simulink library "IPT_lib"  (Simulink 7.4)
settings: Solver=ode45  StartTime=0.0  StopTime=10.0  RelTol=1e-3
values from neighbouring files (symbols this model uses):
  IPTa_i_ShuntCur = mpt.Parameter    [IPT_ANALOG_CAL.m]
  IPTc_Gain_KL30 = mpt.Parameter    [IPT_ANALOG_CAL.m]
  IPTc_Gain_MSDVolt = mpt.Parameter    [IPT_ANALOG_CAL.m]
  IPTc_Gain_PCBTemp = mpt.Parameter    [IPT_ANALOG_CAL.m]
  IPTc_Gain_PosCtrVoltRef1_back = mpt.Parameter    [IPT_ANALOG_CAL.m]
  IPTc_Gain_PosCtrVoltRef1_front = mpt.Parameter    [IPT_ANALOG_CAL.m]
  IPTc_Gain_PosCtrVoltRef2_back = mpt.Parameter    [IPT_ANALOG_CAL.m]
  IPTc_Gain_PosCtrVoltRef2_front = mpt.Parameter    [IPT_ANALOG_CAL.m]
  IPTc_pct_CellInitSoc = mpt.Parameter    [IPT_INTERNAL_CAL.m]
  IPTc_t_BMUInitTemp = mpt.Parameter    [IPT_CAN_CAL.m]
  IPTc_t_MdlInitTemp = mpt.Parameter    [IPT_CAN_CAL.m]
  IPTc_t_PCBTemp_max = mpt.Parameter    [IPT_ANALOG_CAL.m]
  IPTc_t_PCBTemp_min = mpt.Parameter    [IPT_ANALOG_CAL.m]
  IPTc_v_KL30_max = mpt.Parameter    [IPT_ANALOG_CAL.m]
  IPTc_v_KL30_min = mpt.Parameter    [IPT_ANALOG_CAL.m]
  IPTc_v_MSDVolt_max = mpt.Parameter    [IPT_ANALOG_CAL.m]
  IPTc_v_MSDVolt_min = mpt.Parameter    [IPT_ANALOG_CAL.m]
  IPTc_v_PosCtrVoltRef1_back_max = mpt.Parameter    [IPT_ANALOG_CAL.m]
  IPTc_v_PosCtrVoltRef1_back_min = mpt.Parameter    [IPT_ANALOG_CAL.m]
  IPTc_v_PosCtrVoltRef1_front_max = mpt.Parameter    [IPT_ANALOG_CAL.m]
  IPTc_v_PosCtrVoltRef1_front_min = mpt.Parameter    [IPT_ANALOG_CAL.m]
  IPTc_v_PosCtrVoltRef2_back_max = mpt.Parameter    [IPT_ANALOG_CAL.m]
  IPTc_v_PosCtrVoltRef2_back_min = mpt.Parameter    [IPT_ANALOG_CAL.m]
  IPTc_v_PosCtrVoltRef2_front_max = mpt.Parameter    [IPT_ANALOG_CAL.m]
  IPTc_v_PosCtrVoltRef2_front_min = mpt.Parameter    [IPT_ANALOG_CAL.m]
  IPTf_fac_ShuntCurCorrect = mpt.Parameter    [IPT_ANALOG_CAL.m]
undefined symbols (not defined in the file or in its folder): CTC_DriveOnline_St, CTC_FastChaOnline_St, CTC_SlowChaOnline_St, IPTa_v_PCBTemp, IPTc_Gain_BMUPowSplyCur, IPTc_Gain_ShuntCur, IPTc_Gain_USample, IPTc_i_BMUPowSplyCur_max, IPTc_i_BMUPowSplyCur_min, IPTc_i_ShuntCur_max, IPTc_i_ShuntCur_min, IPTc_v_CC2_OffDnLimit, IPTc_v_CC2_OffUpLimit, IPTc_v_CC2_OnDnLimit, IPTc_v_CC2_OnUpLimit, IPTc_v_CellInitVolt, IPTc_v_SlowChalineCnctStLowLimFir, IPTc_v_SlowChalineCnctStLowLimSec, IPTc_v_SlowChalineCnctStUppLimFir, IPTc_v_SlowChalineCnctStUppLimSec, IPTc_v_SlowChalineOpenLowLim, IPTc_v_SlowChalineOpenUppLim, IPTc_v_USample_max, IPTc_v_USample_min, IPTf_t_PCBTemp, PACK_Const_BMUNumOfPack
libraries: Defined_Functionality x129
(part 2 of 3)

== system IPT_lib/IPT/ip_analog/PosCtrVoltRef1_front ==
  HLd_adc_PosCtrVoltRef1_front : Inport
  IPTd_flg_VoltFlterAlwd : Inport  Port=2
  ADC to Actual Value1 : Defined_Functionality/ADC to Actual Value1  SystemSampleTime=-1  offset=IPTc_Offset_PosCtrVoltRef1_front  gain=IPTc_Gain_PosCtrVoltRef1_front
      settings: AttributesFormatString=[OFFSET=%<offset>]\n[GAIN=%<gain>]
  Constant : Constant  Value=IPTc_v_PosCtrVoltRef1_front_max  OutDataTypeMode=single  OutDataType=fixdt(1, 16)  OutScaling=2^0  OutDataTypeStr=single
  Constant1 : Constant  Value=IPTc_v_PosCtrVoltRef1_front_min  OutDataTypeMode=single  OutDataType=fixdt(1, 16)  OutScaling=2^0  OutDataTypeStr=single
  LPF1 : Defined_Functionality/LPF  SystemSampleTime=-1  filter_gain=IPTc_flter_PosCtrVoltRef1_front
      settings: AttributesFormatString=[FILTER_GAIN=%<filter_gain>]
  Logical Operator : Logic  Operator=OR  AllPortsSameDT=off  OutDataTypeMode=boolean  LogicDataType=fixdt(0, 8)  OutDataTypeStr=boolean
  Relational Operator : RelationalOperator  Operator=>  LogicOutDataTypeMode=boolean  LogicDataType=fixdt(0, 8)  OutDataTypeStr=boolean
  Relational Operator1 : RelationalOperator  Operator=<  LogicOutDataTypeMode=boolean  LogicDataType=fixdt(0, 8)  OutDataTypeStr=boolean
  Switch14 : Switch  Criteria=u2 ~= 0  Threshold=0.5  OutDataTypeMode=single  OutDataType=sfix(16)  OutScaling=2^0  OutDataTypeStr=single
  saturation : Defined_Functionality/saturation  SystemSampleTime=-1  upper_limit=IPTc_v_PosCtrVoltRef1_front_max  lower_limit=IPTc_v_PosCtrVoltRef1_front_min
      settings: AttributesFormatString=[UPPER_LIMIT=%<upper_limit>]\n[LOWER_LIMIT=%<lower_limit>]
  signal_debug : Defined_Functionality/signal_debug  SystemSampleTime=-1  debug_switch=IPTc_dbgsw_PosCtrVoltRef1_front  debug_value=IPTc_dbgval_PosCtrVoltRef1_front
  IPTd_v_PosCtrVoltRef1_front : Outport
  IPTd_iflt_PosCtrVoltRef1_front : Outport  Port=2
  wires:
  ADC to Actual Value1/1 -> [IPTd_v_Raw], LPF1/1
  [IPTd_v_Raw] -> Switch14/3
  LPF1/1 -> Switch14/1
  Switch14/1 -> Relational Operator1/1, Relational Operator/1, saturation/1
  IPTd_flg_VoltFlterAlwd/1 -> Switch14/2
  Constant/1 -> Relational Operator/2
  Constant1/1 -> Relational Operator1/2
  Relational Operator/1 -> Logical Operator/1
  Relational Operator1/1 -> Logical Operator/2
  saturation/1 -> signal_debug/1
  HLd_adc_PosCtrVoltRef1_front/1 -> ADC to Actual Value1/1
  Logical Operator/1 -> IPTd_iflt_PosCtrVoltRef1_front/1  "IPTd_iflt_PosCtrVoltRef1_front"
  signal_debug/1 -> IPTd_v_PosCtrVoltRef1_front/1  "IPTd_v_PosCtrVoltRef1_front"

== system IPT_lib/IPT/ip_analog/PosCtrVoltRef2_back ==
  HLd_adc_PosCtrVoltRef2_back : Inport
  IPTd_flg_VoltFlterAlwd : Inport  Port=2
  ADC to Actual Value1 : Defined_Functionality/ADC to Actual Value1  SystemSampleTime=-1  offset=IPTc_Offset_PosCtrVoltRef2_back  gain=IPTc_Gain_PosCtrVoltRef2_back
      settings: AttributesFormatString=[OFFSET=%<offset>]\n[GAIN=%<gain>]
  Constant : Constant  Value=IPTc_v_PosCtrVoltRef2_back_max  OutDataTypeMode=single  OutDataType=fixdt(1, 16)  OutScaling=2^0  OutDataTypeStr=single
  Constant1 : Constant  Value=IPTc_v_PosCtrVoltRef2_back_min  OutDataTypeMode=single  OutDataType=fixdt(1, 16)  OutScaling=2^0  OutDataTypeStr=single
  LPF1 : Defined_Functionality/LPF  SystemSampleTime=-1  filter_gain=IPTc_flter_PosCtrVoltRef2_back
      settings: AttributesFormatString=[FILTER_GAIN=%<filter_gain>]
  Logical Operator : Logic  Operator=OR  AllPortsSameDT=off  OutDataTypeMode=boolean  LogicDataType=fixdt(0, 8)  OutDataTypeStr=boolean
  Relational Operator : RelationalOperator  Operator=>  LogicOutDataTypeMode=boolean  LogicDataType=fixdt(0, 8)  OutDataTypeStr=boolean
  Relational Operator1 : RelationalOperator  Operator=<  LogicOutDataTypeMode=boolean  LogicDataType=fixdt(0, 8)  OutDataTypeStr=boolean
  Switch14 : Switch  Criteria=u2 ~= 0  Threshold=0.5  OutDataTypeMode=single  OutDataType=sfix(16)  OutScaling=2^0  OutDataTypeStr=single
  saturation : Defined_Functionality/saturation  SystemSampleTime=-1  upper_limit=IPTc_v_PosCtrVoltRef2_back_max  lower_limit=IPTc_v_PosCtrVoltRef2_back_min
      settings: AttributesFormatString=[UPPER_LIMIT=%<upper_limit>]\n[LOWER_LIMIT=%<lower_limit>]
  signal_debug : Defined_Functionality/signal_debug  SystemSampleTime=-1  debug_switch=IPTc_dbgsw_PosCtrVoltRef2_back  debug_value=IPTc_dbgval_PosCtrVoltRef2_back
  IPTd_v_PosCtrVoltRef2_back : Outport
  IPTd_iflt_PosCtrVoltRef2_back : Outport  Port=2
  wires:
  ADC to Actual Value1/1 -> [IPTd_v_Raw], LPF1/1  "IPTd_v_PosCtrVoltRef2_back_raw"
  Switch14/1 -> Relational Operator1/1, Relational Operator/1, saturation/1
  LPF1/1 -> Switch14/1
  [IPTd_v_Raw] -> Switch14/3
  IPTd_flg_VoltFlterAlwd/1 -> Switch14/2
  Relational Operator/1 -> Logical Operator/1
  Constant/1 -> Relational Operator/2
  Constant1/1 -> Relational Operator1/2
  Relational Operator1/1 -> Logical Operator/2
  saturation/1 -> signal_debug/1
  HLd_adc_PosCtrVoltRef2_back/1 -> ADC to Actual Value1/1
  Logical Operator/1 -> IPTd_iflt_PosCtrVoltRef2_back/1  "IPTd_iflt_PosCtrVoltRef2_back"
  signal_debug/1 -> IPTd_v_PosCtrVoltRef2_back/1  "IPTd_v_PosCtrVoltRef2_back"

== system IPT_lib/IPT/ip_analog/PosCtrVoltRef2_front ==
  HLd_adc_PosCtrVoltRef2_front : Inport
  IPTd_flg_VoltFlterAlwd : Inport  Port=2
  ADC to Actual Value1 : Defined_Functionality/ADC to Actual Value1  SystemSampleTime=-1  offset=IPTc_Offset_PosCtrVoltRef2_front  gain=IPTc_Gain_PosCtrVoltRef2_front
      settings: AttributesFormatString=[OFFSET=%<offset>]\n[GAIN=%<gain>]
  Constant : Constant  Value=IPTc_v_PosCtrVoltRef2_front_max  OutDataTypeMode=single  OutDataType=fixdt(1, 16)  OutScaling=2^0  OutDataTypeStr=single
  Constant1 : Constant  Value=IPTc_v_PosCtrVoltRef2_front_min  OutDataTypeMode=single  OutDataType=fixdt(1, 16)  OutScaling=2^0  OutDataTypeStr=single
  LPF1 : Defined_Functionality/LPF  SystemSampleTime=-1  filter_gain=IPTc_flter_PosCtrVoltRef2_front
      settings: AttributesFormatString=[FILTER_GAIN=%<filter_gain>]
  Logical Operator : Logic  Operator=OR  AllPortsSameDT=off  OutDataTypeMode=boolean  LogicDataType=fixdt(0, 8)  OutDataTypeStr=boolean
  Relational Operator : RelationalOperator  Operator=>  LogicOutDataTypeMode=boolean  LogicDataType=fixdt(0, 8)  OutDataTypeStr=boolean
  Relational Operator1 : RelationalOperator  Operator=<  LogicOutDataTypeMode=boolean  LogicDataType=fixdt(0, 8)  OutDataTypeStr=boolean
  Switch14 : Switch  Criteria=u2 ~= 0  Threshold=0.5  OutDataTypeMode=single  OutDataType=sfix(16)  OutScaling=2^0  OutDataTypeStr=single
  saturation : Defined_Functionality/saturation  SystemSampleTime=-1  upper_limit=IPTc_v_PosCtrVoltRef2_front_max  lower_limit=IPTc_v_PosCtrVoltRef2_front_min
      settings: AttributesFormatString=[UPPER_LIMIT=%<upper_limit>]\n[LOWER_LIMIT=%<lower_limit>]
  signal_debug : Defined_Functionality/signal_debug  SystemSampleTime=-1  debug_switch=IPTc_dbgsw_PosCtrVoltRef2_front  debug_value=IPTc_dbgval_PosCtrVoltRef2_front
  IPTd_v_PosCtrVoltRef2_front : Outport
  IPTd_iflt_PosCtrVoltRef2_front : Outport  Port=2
  wires:
  ADC to Actual Value1/1 -> [IPTd_v_Raw], LPF1/1  "IPTd_v_PosCtrVoltRef2_front_raw"
  Switch14/1 -> Relational Operator1/1, Relational Operator/1, saturation/1
  LPF1/1 -> Switch14/1
  [IPTd_v_Raw] -> Switch14/3
  IPTd_flg_VoltFlterAlwd/1 -> Switch14/2
  Constant/1 -> Relational Operator/2
  Relational Operator1/1 -> Logical Operator/2
  Relational Operator/1 -> Logical Operator/1
  Constant1/1 -> Relational Operator1/2
  saturation/1 -> signal_debug/1
  signal_debug/1 -> IPTd_v_PosCtrVoltRef2_front/1  "IPTd_v_PosCtrVoltRef2_front"
  Logical Operator/1 -> IPTd_iflt_PosCtrVoltRef2_front/1  "IPTd_iflt_PosCtrVoltRef2_front"
  HLd_adc_PosCtrVoltRef2_front/1 -> ADC to Actual Value1/1

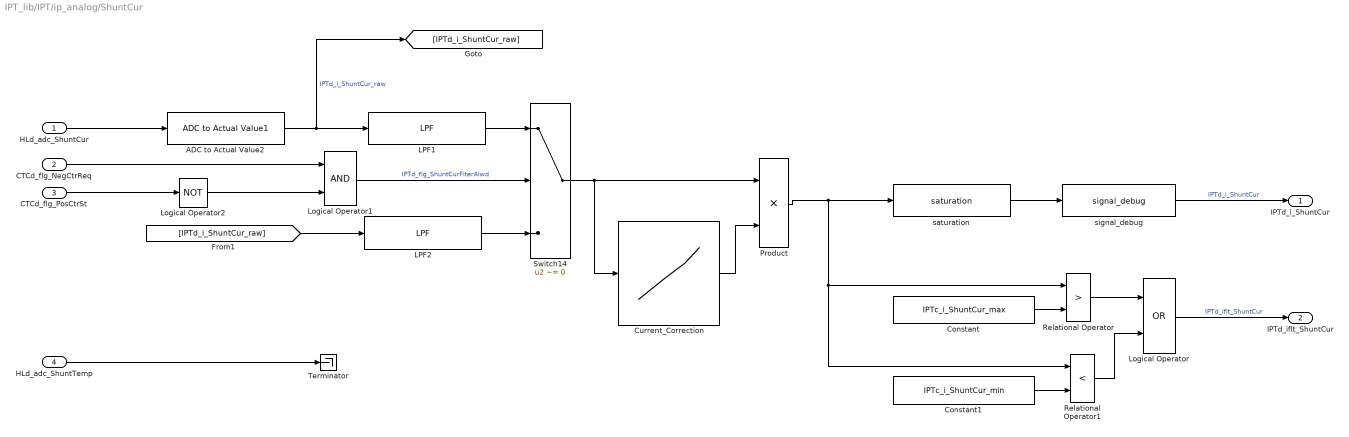
== system IPT_lib/IPT/ip_analog/ShuntCur ==
  HLd_adc_ShuntCur : Inport
  CTCd_flg_NegCtrReq : Inport  Port=2
  CTCd_flg_PosCtrSt : Inport  Port=3
  HLd_adc_ShuntTemp : Inport  Port=4
  ADC to Actual Value2 : Defined_Functionality/ADC to Actual Value1  SystemSampleTime=-1  offset=IPTc_Offset_ShuntCur  gain=IPTc_Gain_ShuntCur
      settings: AttributesFormatString=[OFFSET=%<offset>]\n[GAIN=%<gain>]
  Constant : Constant  Value=IPTc_i_ShuntCur_max  OutDataTypeMode=single  OutDataType=fixdt(1, 16)  OutScaling=2^0  OutDataTypeStr=single
  Constant1 : Constant  Value=IPTc_i_ShuntCur_min  OutDataTypeMode=single  OutDataType=fixdt(1, 16)  OutScaling=2^0  OutDataTypeStr=single
  Current_Correction : Lookup  InputValues=IPTa_i_ShuntCur  Table=IPTf_fac_ShuntCurCorrect  OutDataType=fixdt(1, 16)  OutScaling=2^0
  LPF1 : Defined_Functionality/LPF  SystemSampleTime=-1  filter_gain=IPTc_flter_ShuntCur1
      settings: AttributesFormatString=[FILTER_GAIN=%<filter_gain>]
  LPF2 : Defined_Functionality/LPF  SystemSampleTime=-1  filter_gain=IPTc_flter_ShuntCur2
      settings: AttributesFormatString=[FILTER_GAIN=%<filter_gain>]
  Logical Operator : Logic  Operator=OR  AllPortsSameDT=off  OutDataTypeMode=boolean  LogicDataType=fixdt(0, 8)  OutDataTypeStr=boolean
  Logical Operator1 : Logic  AllPortsSameDT=off  OutDataTypeMode=boolean  LogicDataType=fixdt(0, 8)  OutDataTypeStr=boolean
  Logical Operator2 : Logic  Operator=NOT  AllPortsSameDT=off  OutDataTypeMode=boolean  LogicDataType=fixdt(0, 8)  OutDataTypeStr=boolean
  Product : Product  OutDataType=fixdt(1, 16)  OutScaling=2^0  RndMeth=Zero
  Relational Operator : RelationalOperator  Operator=>  LogicOutDataTypeMode=boolean  LogicDataType=fixdt(0, 8)  OutDataTypeStr=boolean
  Relational Operator1 : RelationalOperator  Operator=<  LogicOutDataTypeMode=boolean  LogicDataType=fixdt(0, 8)  OutDataTypeStr=boolean
  Switch14 : Switch  Criteria=u2 ~= 0  Threshold=0.5  OutDataTypeMode=single  OutDataType=sfix(16)  OutScaling=2^0  OutDataTypeStr=single
  Terminator : Terminator
  saturation : Defined_Functionality/saturation  SystemSampleTime=-1  upper_limit=IPTc_i_ShuntCur_max  lower_limit=IPTc_i_ShuntCur_min
      settings: AttributesFormatString=[UPPER_LIMIT=%<upper_limit>]\n[LOWER_LIMIT=%<lower_limit>]
  signal_debug : Defined_Functionality/signal_debug  SystemSampleTime=-1  debug_switch=IPTc_dbgsw_ShuntCur  debug_value=IPTc_dbgval_ShuntCur
  IPTd_i_ShuntCur : Outport
  IPTd_iflt_ShuntCur : Outport  Port=2
  wires:
  Product/1 -> Relational Operator1/1, Relational Operator/1, saturation/1
  Current_Correction/1 -> Product/2
  Logical Operator2/1 -> Logical Operator1/2
  Logical Operator1/1 -> Switch14/2  "IPTd_flg_ShuntCurFlterAlwd"
  CTCd_flg_PosCtrSt/1 -> Logical Operator2/1
  LPF2/1 -> Switch14/3
  CTCd_flg_NegCtrReq/1 -> Logical Operator1/1
  Switch14/1 -> Current_Correction/1, Product/1
  LPF1/1 -> Switch14/1
  [IPTd_i_ShuntCur_raw] -> LPF2/1
  ADC to Actual Value2/1 -> [IPTd_i_ShuntCur_raw], LPF1/1  "IPTd_i_ShuntCur_raw"
  Constant/1 -> Relational Operator/2
  Relational Operator1/1 -> Logical Operator/2
  Relational Operator/1 -> Logical Operator/1
  Constant1/1 -> Relational Operator1/2
  saturation/1 -> signal_debug/1
  HLd_adc_ShuntTemp/1 -> Terminator/1
  signal_debug/1 -> IPTd_i_ShuntCur/1  "IPTd_i_ShuntCur"
  Logical Operator/1 -> IPTd_iflt_ShuntCur/1  "IPTd_iflt_ShuntCur"
  HLd_adc_ShuntCur/1 -> ADC to Actual Value2/1

== system IPT_lib/IPT/ip_analog/USample ==
  HLd_adc_USample : Inport
  ADC to Actual Value1 : Defined_Functionality/ADC to Actual Value1  SystemSampleTime=-1  offset=IPTc_Offset_USample  gain=IPTc_Gain_USample
      settings: AttributesFormatString=[OFFSET=%<offset>]\n[GAIN=%<gain>]
  Constant : Constant  Value=IPTc_v_USample_max  OutDataTypeMode=single  OutDataType=fixdt(1, 16)  OutScaling=2^0  OutDataTypeStr=single
  Constant1 : Constant  Value=IPTc_v_USample_min  OutDataTypeMode=single  OutDataType=fixdt(1, 16)  OutScaling=2^0  OutDataTypeStr=single
  LPF1 : Defined_Functionality/LPF  SystemSampleTime=-1  filter_gain=IPTc_filter_USample
      settings: AttributesFormatString=[FILTER_GAIN=%<filter_gain>]
  Logical Operator : Logic  Operator=OR  AllPortsSameDT=off  OutDataTypeMode=boolean  LogicDataType=fixdt(0, 8)  OutDataTypeStr=boolean
  Relational Operator : RelationalOperator  Operator=>  LogicOutDataTypeMode=boolean  LogicDataType=fixdt(0, 8)  OutDataTypeStr=boolean
  Relational Operator1 : RelationalOperator  Operator=<  LogicOutDataTypeMode=boolean  LogicDataType=fixdt(0, 8)  OutDataTypeStr=boolean
  saturation : Defined_Functionality/saturation  SystemSampleTime=-1  upper_limit=IPTc_v_USample_max  lower_limit=IPTc_v_USample_min
      settings: AttributesFormatString=[UPPER_LIMIT=%<upper_limit>]\n[LOWER_LIMIT=%<lower_limit>]
  signal_debug1 : Defined_Functionality/signal_debug  SystemSampleTime=-1  debug_switch=IPTc_dbgsw_USample  debug_value=IPTc_dbgval_USample
      settings: AttributesFormatString=[SWITCH=%<debug_switch>]\n[VALUE=%<debug_value>]
  IPTd_v_USample : Outport  DataType=single  OutDataTypeStr=single
  IPTd_iflt_USample : Outport  Port=2
  wires:
  ADC to Actual Value1/1 -> LPF1/1  "IPTd_v_USample_raw"
  LPF1/1 -> Relational Operator1/1, Relational Operator/1, saturation/1
  Constant/1 -> Relational Operator/2
  Constant1/1 -> Relational Operator1/2
  Relational Operator/1 -> Logical Operator/1
  Relational Operator1/1 -> Logical Operator/2
  saturation/1 -> signal_debug1/1
  HLd_adc_USample/1 -> ADC to Actual Value1/1
  Logical Operator/1 -> IPTd_iflt_USample/1  "IPTd_iflt_USample"
  signal_debug1/1 -> IPTd_v_USample/1  "IPTd_v_USample"

== system IPT_lib/IPT/ip_analog/VoltFlterAlwd ==
  CTCd_enum_CtrSt : Inport
  Constant2 : Constant  Value=CTC_DriveOnline_St  OutDataTypeMode=uint8  OutDataType=fixdt(1, 16)  OutScaling=2^0  OutDataTypeStr=uint8
  Constant3 : Constant  Value=CTC_FastChaOnline_St  OutDataTypeMode=uint8  OutDataType=fixdt(1, 16)  OutScaling=2^0  OutDataTypeStr=uint8
  Constant4 : Constant  Value=CTC_SlowChaOnline_St  OutDataTypeMode=uint8  OutDataType=fixdt(1, 16)  OutScaling=2^0  OutDataTypeStr=uint8
  Logical Operator1 : Logic  Operator=OR  Inputs=3  AllPortsSameDT=off  OutDataTypeMode=boolean  LogicDataType=fixdt(0, 8)  OutDataTypeStr=boolean
  Relational Operator2 : RelationalOperator  Operator===  LogicOutDataTypeMode=boolean  LogicDataType=fixdt(0, 8)  OutDataTypeStr=boolean
  Relational Operator3 : RelationalOperator  Operator===  LogicOutDataTypeMode=boolean  LogicDataType=fixdt(0, 8)  OutDataTypeStr=boolean
  Relational Operator4 : RelationalOperator  Operator===  LogicOutDataTypeMode=boolean  LogicDataType=fixdt(0, 8)  OutDataTypeStr=boolean
  debounce : Defined_Functionality/debounce  SystemSampleTime=-1  debounce_time=100
      settings: AttributesFormatString=[DEBOUNCE_TIME=%<debounce_time>]
  IPTd_flg_VoltFlterAlwd : Outport
  wires:
  debounce/1 -> IPTd_flg_VoltFlterAlwd/1  "IPTd_flg_VoltFlterAlwd"
  CTCd_enum_CtrSt/1 -> Relational Operator2/1, Relational Operator3/1, Relational Operator4/1
  Constant2/1 -> Relational Operator2/2
  Constant3/1 -> Relational Operator3/2
  Constant4/1 -> Relational Operator4/2
  Relational Operator2/1 -> Logical Operator1/1
  Relational Operator3/1 -> Logical Operator1/2
  Relational Operator4/1 -> Logical Operator1/3
  Logical Operator1/1 -> debounce/1

== system IPT_lib/IPT/ip_can/BMU_BMS_200ms ==
  HLd_enum_BMUNodeStatus : Inport
  HLd_enum_BMUNmStatus : Inport  Port=2
  HLd_enum_BMUErrorCode : Inport  Port=3
  function : TriggerPort  TriggerType=function-call
  ErrorCode : Subsystem  TreatAsAtomicUnit=on
  NmStatus : Subsystem  TreatAsAtomicUnit=on
  NodeStatus : Subsystem  TreatAsAtomicUnit=on
  IPTd_enum_BMUNodeStatus : Outport
  IPTd_enum_BMUNmStatus : Outport  Port=2
  IPTd_enum_BMUErrorCode : Outport  Port=3
  wires:
  ErrorCode/1(Out) -> IPTd_enum_BMUErrorCode/1  "IPTd_enum_BMUErrorCode"
  NmStatus/1(Out) -> IPTd_enum_BMUNmStatus/1  "IPTd_enum_BMUNmStatus"
  HLd_enum_BMUErrorCode/1 -> ErrorCode/1(In)
  HLd_enum_BMUNmStatus/1 -> NmStatus/1(In)
  HLd_enum_BMUNodeStatus/1 -> NodeStatus/1(In)
  NodeStatus/1(Out) -> IPTd_enum_BMUNodeStatus/1  "IPTd_enum_BMUNodeStatus"

== system IPT_lib/IPT/ip_can/BMU_BMS_300ms ==
  HLd_v_CellVolt : Inport
  function : TriggerPort  TriggerType=function-call
  CellVolt : Subsystem  TreatAsAtomicUnit=on
  MinMax : MinMax  Function=max  OutDataType=fixdt(1, 16)  OutScaling=2^0
  MinMax1 : MinMax  OutDataType=fixdt(1, 16)  OutScaling=2^0
  saturation : Defined_Functionality/saturation  SystemSampleTime=-1  upper_limit=6  lower_limit=0
      settings: AttributesFormatString=[UPPER_LIMIT=%<upper_limit>]\n[LOWER_LIMIT=%<lower_limit>]
  saturation1 : Defined_Functionality/saturation  SystemSampleTime=-1  upper_limit=6  lower_limit=0
      settings: AttributesFormatString=[UPPER_LIMIT=%<upper_limit>]\n[LOWER_LIMIT=%<lower_limit>]
  saturation2 : Defined_Functionality/saturation  SystemSampleTime=-1  upper_limit=6  lower_limit=0
      settings: AttributesFormatString=[UPPER_LIMIT=%<upper_limit>]\n[LOWER_LIMIT=%<lower_limit>]
  signal_debug : Defined_Functionality/signal_debug  SystemSampleTime=-1  debug_switch=IPTc_dbgsw_CellVolt  debug_value=IPTc_dbgval_CellVolt
      settings: AttributesFormatString=[SWITCH=%<debug_switch>]\n[VALUE=%<debug_value>]
  signal_debug1 : Defined_Functionality/signal_debug  SystemSampleTime=-1  debug_switch=IPTc_dbgsw_CellVolt_max  debug_value=IPTc_dbgval_CellVolt_max
      settings: AttributesFormatString=[SWITCH=%<debug_switch>]\n[VALUE=%<debug_value>]
  signal_debug2 : Defined_Functionality/signal_debug  SystemSampleTime=-1  debug_switch=IPTc_dbgsw_CellVolt_min  debug_value=IPTc_dbgval_CellVolt_min
      settings: AttributesFormatString=[SWITCH=%<debug_switch>]\n[VALUE=%<debug_value>]
  IPTd_v_CellVolt : Outport
  IPTd_v_CellVolt_max : Outport  Port=2
  IPTd_v_CellVolt_min : Outport  Port=3
  wires:
  HLd_v_CellVolt/1 -> CellVolt/1(In)
  signal_debug2/1 -> IPTd_v_CellVolt_min/1  "IPTd_v_CellVolt_min"
  signal_debug1/1 -> IPTd_v_CellVolt_max/1  "IPTd_v_CellVolt_max"
  saturation2/1 -> signal_debug2/1
  MinMax1/1 -> saturation2/1
  saturation1/1 -> signal_debug1/1
  MinMax/1 -> saturation1/1
  saturation/1 -> signal_debug/1
  signal_debug/1 -> IPTd_v_CellVolt/1  "IPTd_v_CellVolt"
  CellVolt/1(Out) -> MinMax1/1, MinMax/1, saturation/1

== system IPT_lib/IPT/ip_can/BMU_BMS_500ms ==
  HLd_t_MdlTemp : Inport
  HLd_t_BMUTemp : Inport  Port=2
  function : TriggerPort  TriggerType=function-call
  BMUTemp : Subsystem  TreatAsAtomicUnit=on
  MdlTemp : Subsystem  TreatAsAtomicUnit=on
  saturation : Defined_Functionality/saturation  SystemSampleTime=-1  upper_limit=125  lower_limit=-40
      settings: AttributesFormatString=[UPPER_LIMIT=%<upper_limit>]\n[LOWER_LIMIT=%<lower_limit>]
  saturation1 : Defined_Functionality/saturation  SystemSampleTime=-1  upper_limit=125  lower_limit=-40
      settings: AttributesFormatString=[UPPER_LIMIT=%<upper_limit>]\n[LOWER_LIMIT=%<lower_limit>]
  signal_debug : Defined_Functionality/signal_debug  SystemSampleTime=-1  debug_switch=IPTc_dbgsw_MdlTemp  debug_value=IPTc_dbgval_MdlTemp
      settings: AttributesFormatString=[SWITCH=%<debug_switch>]\n[VALUE=%<debug_value>]
  signal_debug1 : Defined_Functionality/signal_debug  SystemSampleTime=-1  debug_switch=IPTc_dbgsw_BMUTemp  debug_value=IPTc_dbgval_BMUTemp
      settings: AttributesFormatString=[SWITCH=%<debug_switch>]\n[VALUE=%<debug_value>]
  IPTd_t_MdlTemp : Outport
  IPTd_t_BMUTemp : Outport  Port=2
  wires:
  signal_debug1/1 -> IPTd_t_BMUTemp/1  "IPTd_t_BMUTemp"
  saturation1/1 -> signal_debug1/1
  signal_debug/1 -> IPTd_t_MdlTemp/1  "IPTd_t_MdlTemp"
  saturation/1 -> signal_debug/1
  HLd_t_MdlTemp/1 -> MdlTemp/1(In)
  MdlTemp/1(Out) -> saturation/1
  HLd_t_BMUTemp/1 -> BMUTemp/1(In)
  BMUTemp/1(Out) -> saturation1/1

== system IPT_lib/IPT/ip_can/Diagnositc_Enabling ==
  HLd_flg_CANBusOff : Inport
  IPTd_flg_KL15 : Inport  Port=2
  CAN_Bus_Monitoring : Subsystem  RequirementInfo={} %GIDa_5d63c118_d7ad_47c9_a862_cdc8c6015218
  CAN_Diag_Enabling : Subsystem
  IPTd_flg_CANDiagEnable : Outport
  wires:
  CAN_Bus_Monitoring/2(IPTd_cflt_CANBusOff_fault) -> CAN_Diag_Enabling/2(IPTd_cflt_CANBusOff_fault)
  CAN_Bus_Monitoring/1(IPTd_iflt_CANBusOff_fault) -> CAN_Diag_Enabling/1(IPTd_iflt_CANBusOff_fault)
  IPTd_flg_KL15/1 -> CAN_Diag_Enabling/3(IPTd_flg_KL15)
  CAN_Diag_Enabling/1(IPTd_flg_CANDiagEnable) -> IPTd_flg_CANDiagEnable/1
  HLd_flg_CANBusOff/1 -> CAN_Bus_Monitoring/1(HLd_flg_CANBusOff)

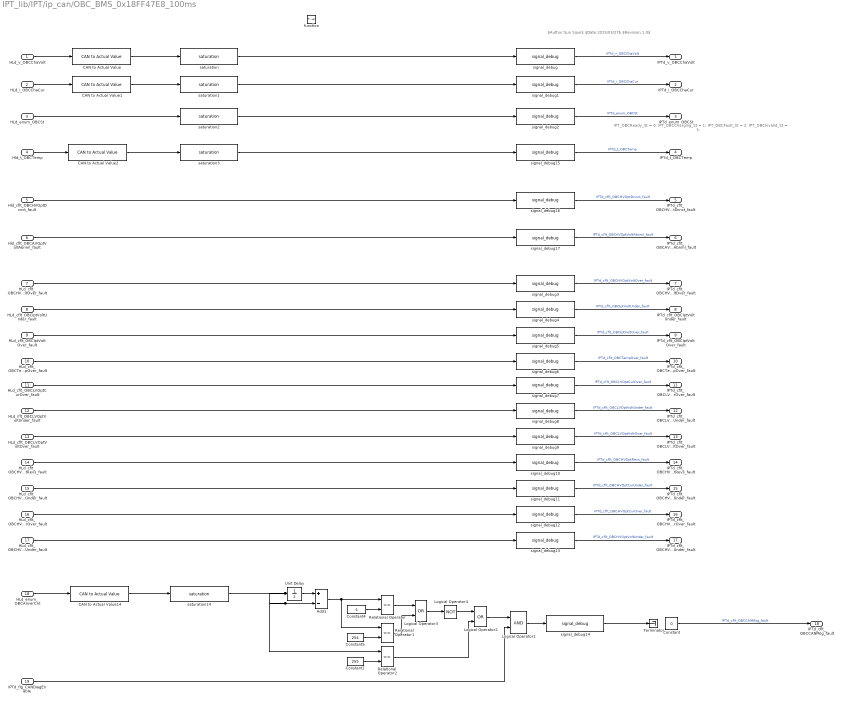
== system IPT_lib/IPT/ip_can/OBC_BMS_0x18FF47E8_100ms ==
  note: IPT_OBCReady_St          = 0;
      | IPT_OBCCharging_St      = 1;
      | IPT_OBCFault_St            = 2;
      | IPT_OBCInvalid_St          = 3;
  note: $Author:Sun Sijun$
      | $Date:2015/03/27$
      | $Revision:1.0$
  HLd_v_OBCChaVolt : Inport
  HLd_i_OBCChaCur : Inport  Port=2
  HLd_enum_OBCSt : Inport  Port=3
  Hld_t_OBCTemp : Inport  Port=4
  Hld_cflt_OBCHVOptDcnct_fault : Inport  Port=5
  Hld_cflt_OBCAVOptVoltAbnml_fault : Inport  Port=6
  HLd_cflt_OBCHVOptVoltOver_fault : Inport  Port=7
  HLd_cflt_OBCIptVoltUnder_fault : Inport  Port=8
  HLd_cflt_OBCIptVoltOver_fault : Inport  Port=9
  HLd_cflt_OBCTempOver_fault : Inport  Port=10
  HLd_cflt_OBCLVOptCurOver_fault : Inport  Port=11
  HLd_iflt_OBCLVOptVoltUnder_fault : Inport  Port=12
  HLd_cflt_OBCLVOptVoltOver_fault : Inport  Port=13
  HLd_cflt_OBCHVOptRevs_fault : Inport  Port=14
  HLd_cflt_OBCHVOptCurUnder_fault : Inport  Port=15
  HLd_cflt_OBCHVOptCurOver_fault : Inport  Port=16
  HLd_cflt_OBCHVOptVoltUnder_fault : Inport  Port=17
  HLd_enum_OBCAliverCnt : Inport  Port=18
  IPTd_flg_CANDiagEnable : Inport  Port=19
  function : TriggerPort  TriggerType=function-call
  Add1 : Sum  Inputs=+-  OutDataTypeMode=int16  OutDataTypeStr=int16
  CAN to Actual Value : Defined_Functionality/CAN to Actual Value  SystemSampleTime=-1  gain=0.1  offset=0
      settings: AttributesFormatString=[GAIN=%<gain>]\n[OFFSET=%<offset>]
  CAN to Actual Value1 : Defined_Functionality/CAN to Actual Value  SystemSampleTime=-1  gain=0.1  offset=0
      settings: AttributesFormatString=[GAIN=%<gain>]\n[OFFSET=%<offset>]
  CAN to Actual Value14 : Defined_Functionality/CAN to Actual Value  SystemSampleTime=-1  gain=1  offset=0
      settings: AttributesFormatString=[GAIN=%<gain>]\n[OFFSET=%<offset>]
  CAN to Actual Value2 : Defined_Functionality/CAN to Actual Value  SystemSampleTime=-1  gain=1  offset=-40
      settings: AttributesFormatString=[GAIN=%<gain>]\n[OFFSET=%<offset>]
  Constant : Constant  Value=0  OutDataTypeMode=boolean  OutDataType=fixdt(1, 16)  OutScaling=2^0  OutDataTypeStr=boolean
  Constant1 : Constant  Value=255  OutDataTypeMode=uint8  OutDataTypeStr=uint8
  Constant4 : Constant  Value=-1  OutDataTypeMode=int8  OutDataTypeStr=int8
  Constant5 : Constant  Value=254  OutDataTypeMode=uint8  OutDataTypeStr=uint8
  Logical Operator1 : Logic  AllPortsSameDT=off  OutDataTypeMode=boolean  LogicDataType=fixdt(0, 8)  OutDataTypeStr=boolean
  Logical Operator2 : Logic  Operator=OR  AllPortsSameDT=off  OutDataTypeMode=boolean  LogicDataType=fixdt(0, 8)  OutDataTypeStr=boolean
  Logical Operator3 : Logic  Operator=OR  AllPortsSameDT=off  OutDataTypeMode=boolean  LogicDataType=fixdt(0, 8)  OutDataTypeStr=boolean
  Logical Operator4 : Logic  Operator=NOT  AllPortsSameDT=off  OutDataTypeMode=boolean  LogicDataType=fixdt(0, 8)  OutDataTypeStr=boolean
  Relational Operator : RelationalOperator  Operator===  LogicOutDataTypeMode=boolean  OutDataTypeStr=boolean
  Relational Operator1 : RelationalOperator  Operator===  LogicOutDataTypeMode=boolean  OutDataTypeStr=boolean
  Relational Operator2 : RelationalOperator  Operator===  LogicOutDataTypeMode=boolean  OutDataTypeStr=boolean
  Terminator : Terminator
  Unit Delay : UnitDelay  SampleTime=-1
  saturation : Defined_Functionality/saturation  SystemSampleTime=-1  upper_limit=660  lower_limit=0
      settings: AttributesFormatString=[UPPER_LIMIT=%<upper_limit>]\n[LOWER_LIMIT=%<lower_limit>]
  saturation1 : Defined_Functionality/saturation  SystemSampleTime=-1  upper_limit=30  lower_limit=0
      settings: AttributesFormatString=[UPPER_LIMIT=%<upper_limit>]\n[LOWER_LIMIT=%<lower_limit>]
  saturation14 : Defined_Functionality/saturation  SystemSampleTime=-1  upper_limit=255  lower_limit=0
      settings: AttributesFormatString=[UPPER_LIMIT=%<upper_limit>]\n[LOWER_LIMIT=%<lower_limit>]
  saturation2 : Defined_Functionality/saturation  SystemSampleTime=-1  upper_limit=3  lower_limit=0
      settings: AttributesFormatString=[UPPER_LIMIT=%<upper_limit>]\n[LOWER_LIMIT=%<lower_limit>]
  saturation3 : Defined_Functionality/saturation  SystemSampleTime=-1  upper_limit=215  lower_limit=-40
      settings: AttributesFormatString=[UPPER_LIMIT=%<upper_limit>]\n[LOWER_LIMIT=%<lower_limit>]
  signal_debug : Defined_Functionality/signal_debug  SystemSampleTime=-1  debug_switch=IPTc_dbgsw_OBCChaVolt  debug_value=IPTc_dbgval_OBCChaVolt
      settings: AttributesFormatString=[SWITCH=%<debug_switch>]\n[VALUE=%<debug_value>]
  signal_debug1 : Defined_Functionality/signal_debug  SystemSampleTime=-1  debug_switch=IPTc_dbgsw_OBCChaCur  debug_value=IPTc_dbgval_OBCChaCur
      settings: AttributesFormatString=[SWITCH=%<debug_switch>]\n[VALUE=%<debug_value>]
  signal_debug10 : Defined_Functionality/signal_debug  SystemSampleTime=-1  debug_switch=IPTc_dbgsw_OBCHVOptRevs_fault  debug_value=IPTc_dbgval_OBCHVOptRevs_fault
      settings: AttributesFormatString=[SWITCH=%<debug_switch>]\n[VALUE=%<debug_value>]
  signal_debug11 : Defined_Functionality/signal_debug  SystemSampleTime=-1  debug_switch=IPTc_dbgsw_OBCHVOptCurUnder_fault  debug_value=IPTc_dbgval_OBCHVOptCurUnder_fault
      settings: AttributesFormatString=[SWITCH=%<debug_switch>]\n[VALUE=%<debug_value>]
  signal_debug12 : Defined_Functionality/signal_debug  SystemSampleTime=-1  debug_switch=IPTc_dbgsw_OBCHVOptCurOver_fault  debug_value=IPTc_dbgval_OBCHVOptCurOver_fault
      settings: AttributesFormatString=[SWITCH=%<debug_switch>]\n[VALUE=%<debug_value>]
  signal_debug13 : Defined_Functionality/signal_debug  SystemSampleTime=-1  debug_switch=IPTc_dbgsw_OBCHVOptVoltUnder_fault  debug_value=IPTc_dbgval_OBCHVOptVoltUnder_fault
      settings: AttributesFormatString=[SWITCH=%<debug_switch>]\n[VALUE=%<debug_value>]
  signal_debug14 : Defined_Functionality/signal_debug  SystemSampleTime=-1  debug_switch=0  debug_value=1
      settings: AttributesFormatString=[SWITCH=%<debug_switch>]\n[VALUE=%<debug_value>]
  signal_debug15 : Defined_Functionality/signal_debug  SystemSampleTime=-1  debug_switch=IPTc_dbgsw_OBCTemp  debug_value=IPTc_dbgval_OBCTemp
      settings: AttributesFormatString=[SWITCH=%<debug_switch>]\n[VALUE=%<debug_value>]
  signal_debug16 : Defined_Functionality/signal_debug  SystemSampleTime=-1  debug_switch=IPTc_dbgsw_OBCHVOptDcnct_fault  debug_value=IPTc_dbgval_OBCHVOptDcnct_fault
      settings: AttributesFormatString=[SWITCH=%<debug_switch>]\n[VALUE=%<debug_value>]
  signal_debug17 : Defined_Functionality/signal_debug  SystemSampleTime=-1  debug_switch=IPTc_dbgsw_OBCAVOptVoltAbnml_fault  debug_value=IPTc_dbgval_OBCAVOptVoltAbnml_fault
      settings: AttributesFormatString=[SWITCH=%<debug_switch>]\n[VALUE=%<debug_value>]
  signal_debug2 : Defined_Functionality/signal_debug  SystemSampleTime=-1  debug_switch=IPTc_dbgsw_OBCSt  debug_value=IPTc_dbgval_OBCSt
      settings: AttributesFormatString=[SWITCH=%<debug_switch>]\n[VALUE=%<debug_value>]
  signal_debug3 : Defined_Functionality/signal_debug  SystemSampleTime=-1  debug_switch=IPTc_dbgsw_OBCHVOptVoltOver_fault  debug_value=IPTc_dbgval_OBCHVOptVoltOver_fault
      settings: AttributesFormatString=[SWITCH=%<debug_switch>]\n[VALUE=%<debug_value>]
  signal_debug4 : Defined_Functionality/signal_debug  SystemSampleTime=-1  debug_switch=IPTc_dbgsw_OBCIptVoltUnder_fault  debug_value=IPTc_dbgval_OBCIptVoltUnder_fault
      settings: AttributesFormatString=[SWITCH=%<debug_switch>]\n[VALUE=%<debug_value>]
  signal_debug5 : Defined_Functionality/signal_debug  SystemSampleTime=-1  debug_switch=IPTc_dbgsw_OBCIptVoltOver_fault  debug_value=IPTc_dbgval_OBCIptVoltOver_fault
      settings: AttributesFormatString=[SWITCH=%<debug_switch>]\n[VALUE=%<debug_value>]
  signal_debug6 : Defined_Functionality/signal_debug  SystemSampleTime=-1  debug_switch=IPTc_dbgsw_OBCTempOver_fault  debug_value=IPTc_dbgval_OBCTempOver_fault
      settings: AttributesFormatString=[SWITCH=%<debug_switch>]\n[VALUE=%<debug_value>]
  signal_debug7 : Defined_Functionality/signal_debug  SystemSampleTime=-1  debug_switch=IPTc_dbgsw_OBCLVOptCurOver_fault  debug_value=IPTc_dbgval_OBCLVOptCurOver_fault
      settings: AttributesFormatString=[SWITCH=%<debug_switch>]\n[VALUE=%<debug_value>]
  signal_debug8 : Defined_Functionality/signal_debug  SystemSampleTime=-1  debug_switch=IPTc_dbgsw_OBCLVOptVoltUnder_fault  debug_value=IPTc_dbgval_OBCLVOptVoltUnder_fault
      settings: AttributesFormatString=[SWITCH=%<debug_switch>]\n[VALUE=%<debug_value>]
  signal_debug9 : Defined_Functionality/signal_debug  SystemSampleTime=-1  debug_switch=IPTc_dbgsw_OBCLVOptVoltOver_fault  debug_value=IPTc_dbgval_OBCLVOptVoltOver_fault
      settings: AttributesFormatString=[SWITCH=%<debug_switch>]\n[VALUE=%<debug_value>]
  IPTd_v_OBCChaVolt : Outport
  IPTd_i_OBCChaCur : Outport  Port=2
  IPTd_enum_OBCSt : Outport  Port=3
  IPTd_t_OBCTemp : Outport  Port=4
  IPTd_cflt_OBCHVOptDcnct_fault : Outport  Port=5
  IPTd_cflt_OBCAVOptVoltAbnml_fault : Outport  Port=6
  IPTd_cflt_OBCHVOptVoltOver_fault : Outport  Port=7
  IPTd_cflt_OBCIptVoltUnder_fault : Outport  Port=8
  IPTd_cflt_OBCIptVoltOver_fault : Outport  Port=9
  IPTd_cflt_OBCTempOver_fault : Outport  Port=10
  IPTd_cflt_OBCLVOptCurOver_fault : Outport  Port=11
  IPTd_cflt_OBCLVOptVoltUnder_fault : Outport  Port=12
  IPTd_cflt_OBCLVOptVoltOver_fault : Outport  Port=13
  IPTd_cflt_OBCHVOptRevs_fault : Outport  Port=14
  IPTd_cflt_OBCHVOptCurUnder_fault : Outport  Port=15
  IPTd_cflt_OBCHVOptCurOver_fault : Outport  Port=16
  IPTd_cflt_OBCHVOptVoltUnder_fault : Outport  Port=17
  IPTd_cflt_OBCCANMsg_fault : Outport  Port=18  InitialOutput=0
  wires:
  signal_debug17/1 -> IPTd_cflt_OBCAVOptVoltAbnml_fault/1  "IPTd_cflt_OBCAVOptVoltAbnml_fault"
  signal_debug16/1 -> IPTd_cflt_OBCHVOptDcnct_fault/1  "IPTd_cflt_OBCHVOptDcnct_fault"
  Hld_cflt_OBCAVOptVoltAbnml_fault/1 -> signal_debug17/1
  Hld_cflt_OBCHVOptDcnct_fault/1 -> signal_debug16/1
  signal_debug15/1 -> IPTd_t_OBCTemp/1  "IPTd_t_OBCTemp"
  saturation3/1 -> signal_debug15/1
  CAN to Actual Value2/1 -> saturation3/1
  Hld_t_OBCTemp/1 -> CAN to Actual Value2/1
  Constant/1 -> IPTd_cflt_OBCCANMsg_fault/1  "IPTd_cflt_OBCCANMsg_fault"
  Logical Operator2/1 -> Logical Operator1/1
  Relational Operator2/1 -> Logical Operator2/2
  Logical Operator4/1 -> Logical Operator2/1
  Logical Operator3/1 -> Logical Operator4/1
  Constant1/1 -> Relational Operator2/2
  Relational Operator1/1 -> Logical Operator3/2
  Relational Operator/1 -> Logical Operator3/1
  Add1/1 -> Relational Operator1/1, Relational Operator/1
  Unit Delay/1 -> Add1/1
  Constant4/1 -> Relational Operator/2
  Constant5/1 -> Relational Operator1/2
  saturation14/1 -> Relational Operator2/1, Add1/2, Unit Delay/1
  Logical Operator1/1 -> signal_debug14/1
  CAN to Actual Value14/1 -> saturation14/1
  HLd_cflt_OBCLVOptVoltOver_fault/1 -> signal_debug9/1
  signal_debug9/1 -> IPTd_cflt_OBCLVOptVoltOver_fault/1  "IPTd_cflt_OBCLVOptVoltOver_fault"
  signal_debug14/1 -> Terminator/1
  signal_debug13/1 -> IPTd_cflt_OBCHVOptVoltUnder_fault/1  "IPTd_cflt_OBCHVOptVoltUnder_fault"
  signal_debug12/1 -> IPTd_cflt_OBCHVOptCurOver_fault/1  "IPTd_cflt_OBCHVOptCurOver_fault"
  signal_debug11/1 -> IPTd_cflt_OBCHVOptCurUnder_fault/1  "IPTd_cflt_OBCHVOptCurUnder_fault"
  signal_debug10/1 -> IPTd_cflt_OBCHVOptRevs_fault/1  "IPTd_cflt_OBCHVOptRevs_fault"
  signal_debug8/1 -> IPTd_cflt_OBCLVOptVoltUnder_fault/1  "IPTd_cflt_OBCLVOptVoltUnder_fault"
  signal_debug7/1 -> IPTd_cflt_OBCLVOptCurOver_fault/1  "IPTd_cflt_OBCLVOptCurOver_fault"
  signal_debug6/1 -> IPTd_cflt_OBCTempOver_fault/1  "IPTd_cflt_OBCTempOver_fault"
  signal_debug5/1 -> IPTd_cflt_OBCIptVoltOver_fault/1  "IPTd_cflt_OBCIptVoltOver_fault"
  signal_debug4/1 -> IPTd_cflt_OBCIptVoltUnder_fault/1  "IPTd_cflt_OBCIptVoltUnder_fault"
  signal_debug3/1 -> IPTd_cflt_OBCHVOptVoltOver_fault/1  "IPTd_cflt_OBCHVOptVoltOver_fault"
  signal_debug2/1 -> IPTd_enum_OBCSt/1  "IPTd_enum_OBCSt"
  signal_debug1/1 -> IPTd_i_OBCChaCur/1  "IPTd_i_OBCChaCur"
  signal_debug/1 -> IPTd_v_OBCChaVolt/1  "IPTd_v_OBCChaVolt"
  IPTd_flg_CANDiagEnable/1 -> Logical Operator1/2
  saturation2/1 -> signal_debug2/1
  HLd_enum_OBCAliverCnt/1 -> CAN to Actual Value14/1
  HLd_cflt_OBCHVOptVoltUnder_fault/1 -> signal_debug13/1
  HLd_cflt_OBCHVOptCurOver_fault/1 -> signal_debug12/1
  HLd_cflt_OBCHVOptCurUnder_fault/1 -> signal_debug11/1
  HLd_cflt_OBCHVOptRevs_fault/1 -> signal_debug10/1
  HLd_iflt_OBCLVOptVoltUnder_fault/1 -> signal_debug8/1
  HLd_cflt_OBCLVOptCurOver_fault/1 -> signal_debug7/1
  HLd_cflt_OBCTempOver_fault/1 -> signal_debug6/1
  HLd_cflt_OBCIptVoltOver_fault/1 -> signal_debug5/1
  HLd_cflt_OBCIptVoltUnder_fault/1 -> signal_debug4/1
  HLd_enum_OBCSt/1 -> saturation2/1
  HLd_cflt_OBCHVOptVoltOver_fault/1 -> signal_debug3/1
  saturation1/1 -> signal_debug1/1
  HLd_i_OBCChaCur/1 -> CAN to Actual Value1/1
  CAN to Actual Value1/1 -> saturation1/1
  saturation/1 -> signal_debug/1
  CAN to Actual Value/1 -> saturation/1
  HLd_v_OBCChaVolt/1 -> CAN to Actual Value/1

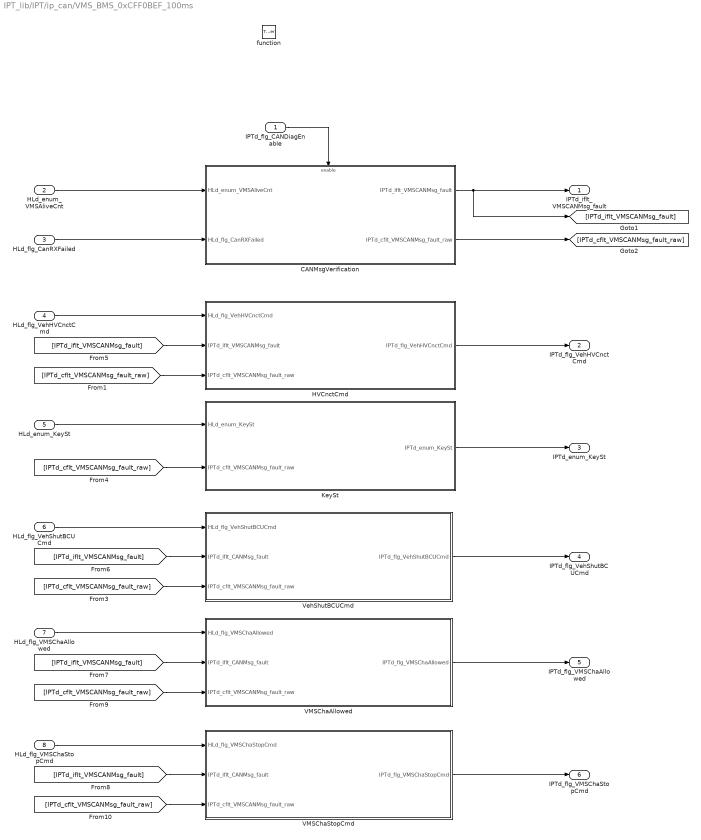
== system IPT_lib/IPT/ip_can/VMS_BMS_0xCFF0BEF_100ms ==
  IPTd_flg_CANDiagEnable : Inport  OutDataType=fixdt(1, 16)  OutScaling=2^0
  HLd_enum_VMSAliveCnt : Inport  Port=2  OutDataType=fixdt(1, 16)  OutScaling=2^0
  HLd_flg_CanRXFailed : Inport  Port=3  OutDataType=fixdt(1, 16)  OutScaling=2^0
  HLd_flg_VehHVCnctCmd : Inport  Port=4  OutDataType=fixdt(1, 16)  OutScaling=2^0
  HLd_enum_KeySt : Inport  Port=5  OutDataType=fixdt(1, 16)  OutScaling=2^0
  HLd_flg_VehShutBCUCmd : Inport  Port=6  OutDataType=fixdt(1, 16)  OutScaling=2^0
  HLd_flg_VMSChaAllowed : Inport  Port=7  OutDataType=fixdt(1, 16)  OutScaling=2^0
  HLd_flg_VMSChaStopCmd : Inport  Port=8  OutDataType=fixdt(1, 16)  OutScaling=2^0
  function : TriggerPort  TriggerType=function-call
  CANMsgVerification : Subsystem
  HVCnctCmd : Subsystem
  KeySt : Subsystem
  VMSChaAllowed : Subsystem
  VMSChaStopCmd : Subsystem
  VehShutBCUCmd : Subsystem
  IPTd_iflt_VMSCANMsg_fault : Outport  OutDataType=fixdt(1, 16)  OutScaling=2^0
  IPTd_flg_VehHVCnctCmd : Outport  Port=2  OutDataType=fixdt(1, 16)  OutScaling=2^0
  IPTd_enum_KeySt : Outport  Port=3  OutDataType=fixdt(1, 16)  OutScaling=2^0
  IPTd_flg_VehShutBCUCmd : Outport  Port=4  OutDataType=fixdt(1, 16)  OutScaling=2^0
  IPTd_flg_VMSChaAllowed : Outport  Port=5  OutDataType=fixdt(1, 16)  OutScaling=2^0
  IPTd_flg_VMSChaStopCmd : Outport  Port=6  OutDataType=fixdt(1, 16)  OutScaling=2^0
  wires:
  HLd_enum_KeySt/1 -> KeySt/1(HLd_enum_KeySt)
  HLd_flg_VehShutBCUCmd/1 -> VehShutBCUCmd/1(HLd_flg_VehShutBCUCmd)
  KeySt/1(IPTd_enum_KeySt) -> IPTd_enum_KeySt/1
  VehShutBCUCmd/1(IPTd_flg_VehShutBCUCmd) -> IPTd_flg_VehShutBCUCmd/1
  VMSChaAllowed/1(IPTd_flg_VMSChaAllowed) -> IPTd_flg_VMSChaAllowed/1
  VMSChaStopCmd/1(IPTd_flg_VMSChaStopCmd) -> IPTd_flg_VMSChaStopCmd/1
  HVCnctCmd/1(IPTd_flg_VehHVCnctCmd) -> IPTd_flg_VehHVCnctCmd/1
  HLd_flg_VMSChaStopCmd/1 -> VMSChaStopCmd/1(HLd_flg_VMSChaStopCmd)
  [IPTd_cflt_VMSCANMsg_fault_raw] -> KeySt/2(IPTd_cflt_VMSCANMsg_fault_raw)
  HLd_flg_VehHVCnctCmd/1 -> HVCnctCmd/1(HLd_flg_VehHVCnctCmd)
  [IPTd_iflt_VMSCANMsg_fault] -> HVCnctCmd/2(IPTd_iflt_VMSCANMsg_fault)
  [IPTd_iflt_VMSCANMsg_fault] -> VehShutBCUCmd/2(IPTd_iflt_CANMsg_fault)
  HLd_flg_VMSChaAllowed/1 -> VMSChaAllowed/1(HLd_flg_VMSChaAllowed)
  [IPTd_iflt_VMSCANMsg_fault] -> VMSChaAllowed/2(IPTd_iflt_CANMsg_fault)
  [IPTd_iflt_VMSCANMsg_fault] -> VMSChaStopCmd/2(IPTd_iflt_CANMsg_fault)
  HLd_enum_VMSAliveCnt/1 -> CANMsgVerification/1(HLd_enum_VMSAliveCnt)
  CANMsgVerification/1(IPTd_iflt_VMSCANMsg_fault) -> IPTd_iflt_VMSCANMsg_fault/1, [IPTd_iflt_VMSCANMsg_fault]
  IPTd_flg_CANDiagEnable/1 -> CANMsgVerification/Enable
  HLd_flg_CanRXFailed/1 -> CANMsgVerification/2(HLd_flg_CanRXFailed)
  CANMsgVerification/2(IPTd_cflt_VMSCANMsg_fault_raw) -> [IPTd_cflt_VMSCANMsg_fault_raw]
  [IPTd_cflt_VMSCANMsg_fault_raw] -> HVCnctCmd/3(IPTd_cflt_VMSCANMsg_fault_raw)
  [IPTd_cflt_VMSCANMsg_fault_raw] -> VehShutBCUCmd/3(IPTd_cflt_VMSCANMsg_fault_raw)
  [IPTd_cflt_VMSCANMsg_fault_raw] -> VMSChaAllowed/3(IPTd_cflt_VMSCANMsg_fault_raw)
  [IPTd_cflt_VMSCANMsg_fault_raw] -> VMSChaStopCmd/3(IPTd_cflt_VMSCANMsg_fault_raw)

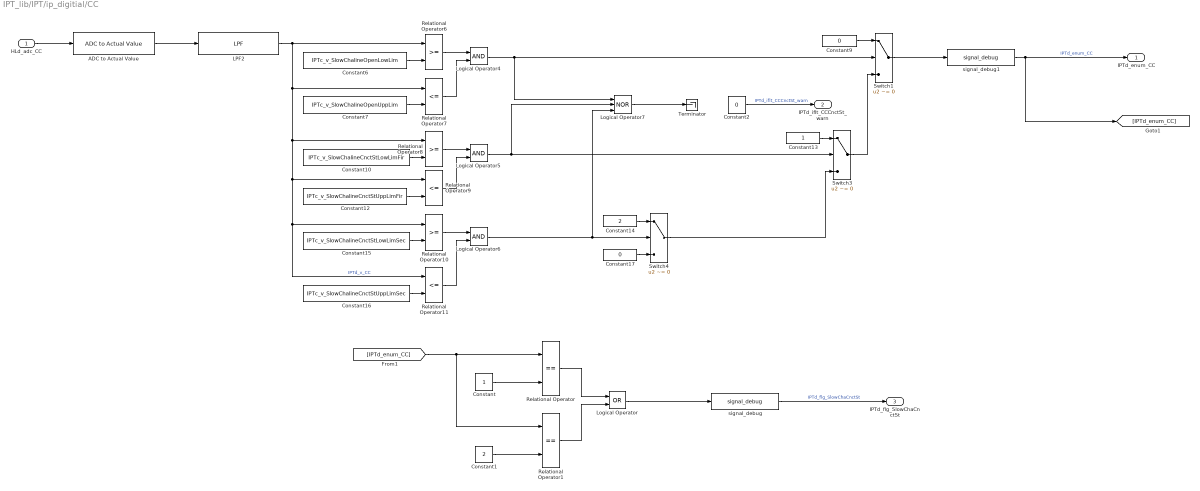
== system IPT_lib/IPT/ip_digitial/CC ==
  HLd_adc_CC : Inport  OutDataType=fixdt(1, 16)  OutScaling=2^0
  ADC to Actual Value : Defined_Functionality/ADC to Actual Value  SystemSampleTime=-1  gain=0.001221  offset=0
      settings: AttributesFormatString=[GAIN=%<gain>]\n[OFFSET=%<offset>]
  Constant : Constant  OutDataTypeMode=uint8  OutDataType=fixdt(1, 16)  OutScaling=2^0  OutDataTypeStr=uint8
  Constant1 : Constant  Value=2  OutDataTypeMode=uint8  OutDataType=fixdt(1, 16)  OutScaling=2^0  OutDataTypeStr=uint8
  Constant10 : Constant  Value=IPTc_v_SlowChalineCnctStLowLimFir  OutDataType=fixdt(1, 16)  OutScaling=2^0
  Constant12 : Constant  Value=IPTc_v_SlowChalineCnctStUppLimFir  OutDataType=fixdt(1, 16)  OutScaling=2^0
  Constant13 : Constant  OutDataTypeMode=uint8  OutDataType=fixdt(1, 16)  OutScaling=2^0  OutDataTypeStr=uint8
  Constant14 : Constant  Value=2  OutDataTypeMode=uint8  OutDataType=fixdt(1, 16)  OutScaling=2^0  OutDataTypeStr=uint8
  Constant15 : Constant  Value=IPTc_v_SlowChalineCnctStLowLimSec  OutDataType=fixdt(1, 16)  OutScaling=2^0
  Constant16 : Constant  Value=IPTc_v_SlowChalineCnctStUppLimSec  OutDataType=fixdt(1, 16)  OutScaling=2^0
  Constant17 : Constant  Value=0  OutDataTypeMode=uint8  OutDataType=fixdt(1, 16)  OutScaling=2^0  OutDataTypeStr=uint8
  Constant2 : Constant  Value=0  OutDataTypeMode=boolean  OutDataType=fixdt(1, 16)  OutScaling=2^0  OutDataTypeStr=boolean
  Constant6 : Constant  Value=IPTc_v_SlowChalineOpenLowLim  OutDataType=fixdt(1, 16)  OutScaling=2^0
  Constant7 : Constant  Value=IPTc_v_SlowChalineOpenUppLim  OutDataType=fixdt(1, 16)  OutScaling=2^0
  Constant9 : Constant  Value=0  OutDataTypeMode=uint8  OutDataType=fixdt(1, 16)  OutScaling=2^0  OutDataTypeStr=uint8
  LPF2 : Defined_Functionality/LPF  SystemSampleTime=-1  filter_gain=1
      settings: AttributesFormatString=[FILTER_GAIN=%<filter_gain>]
  Logical Operator : Logic  Operator=OR  AllPortsSameDT=off  OutDataTypeMode=boolean  LogicDataType=fixdt(0, 8)  OutDataTypeStr=boolean
  Logical Operator4 : Logic  AllPortsSameDT=off  OutDataTypeMode=boolean  LogicDataType=fixdt(0, 8)  OutDataTypeStr=boolean
  Logical Operator5 : Logic  AllPortsSameDT=off  OutDataTypeMode=boolean  LogicDataType=fixdt(0, 8)  OutDataTypeStr=boolean
  Logical Operator6 : Logic  AllPortsSameDT=off  OutDataTypeMode=boolean  LogicDataType=fixdt(0, 8)  OutDataTypeStr=boolean
  Logical Operator7 : Logic  Operator=NOR  Inputs=3  AllPortsSameDT=off  OutDataTypeMode=boolean  LogicDataType=fixdt(0, 8)  OutDataTypeStr=boolean
  Relational Operator : RelationalOperator  Operator===  LogicOutDataTypeMode=boolean  LogicDataType=fixdt(0, 8)  OutDataTypeStr=boolean
  Relational Operator1 : RelationalOperator  Operator===  LogicOutDataTypeMode=boolean  LogicDataType=fixdt(0, 8)  OutDataTypeStr=boolean
  Relational Operator10 : RelationalOperator  LogicOutDataTypeMode=boolean  LogicDataType=fixdt(0, 8)  OutDataTypeStr=boolean
  Relational Operator11 : RelationalOperator  Operator=<=  LogicOutDataTypeMode=boolean  LogicDataType=fixdt(0, 8)  OutDataTypeStr=boolean
  Relational Operator6 : RelationalOperator  LogicOutDataTypeMode=boolean  LogicDataType=fixdt(0, 8)  OutDataTypeStr=boolean
  Relational Operator7 : RelationalOperator  Operator=<=  LogicOutDataTypeMode=boolean  LogicDataType=fixdt(0, 8)  OutDataTypeStr=boolean
  Relational Operator8 : RelationalOperator  LogicOutDataTypeMode=boolean  LogicDataType=fixdt(0, 8)  OutDataTypeStr=boolean
  Relational Operator9 : RelationalOperator  Operator=<=  LogicOutDataTypeMode=boolean  LogicDataType=fixdt(0, 8)  OutDataTypeStr=boolean
  Switch1 : Switch  Criteria=u2 ~= 0  OutDataType=fixdt(1, 16)  OutScaling=2^0
  Switch3 : Switch  Criteria=u2 ~= 0  OutDataType=fixdt(1, 16)  OutScaling=2^0
  Switch4 : Switch  Criteria=u2 ~= 0  OutDataType=fixdt(1, 16)  OutScaling=2^0
  Terminator : Terminator
  signal_debug : Defined_Functionality/signal_debug  SystemSampleTime=-1  debug_switch=IPTc_dbgsw_SlowChaCnctSt  debug_value=IPTc_dbgval_SlowChaCnctSt
      settings: AttributesFormatString=[SWITCH=%<debug_switch>]\n[VALUE=%<debug_value>]
  signal_debug1 : Defined_Functionality/signal_debug  SystemSampleTime=-1  debug_switch=IPTc_dbgsw_CC  debug_value=IPTc_dbgval_CC
      settings: AttributesFormatString=[SWITCH=%<debug_switch>]\n[VALUE=%<debug_value>]
  IPTd_enum_CC : Outport  OutDataType=fixdt(1, 16)  OutScaling=2^0
  IPTd_iflt_CCCnctSt_warn : Outport  Port=2  OutDataType=fixdt(1, 16)  OutScaling=2^0
  IPTd_flg_SlowChaCnctSt : Outport  Port=3  OutDataType=fixdt(1, 16)  OutScaling=2^0
  wires:
  [IPTd_enum_CC] -> Relational Operator1/1, Relational Operator/1
  Logical Operator/1 -> signal_debug/1
  Relational Operator1/1 -> Logical Operator/2
  Relational Operator/1 -> Logical Operator/1
  Constant/1 -> Relational Operator/2
  Constant1/1 -> Relational Operator1/2
  Constant17/1 -> Switch4/3
  Switch4/1 -> Switch3/3
  Constant14/1 -> Switch4/1
  Logical Operator6/1 -> Logical Operator7/3, Switch4/2
  Relational Operator10/1 -> Logical Operator6/1
  Relational Operator11/1 -> Logical Operator6/2
  Constant16/1 -> Relational Operator11/2
  Constant15/1 -> Relational Operator10/2
  Switch3/1 -> Switch1/3
  Constant13/1 -> Switch3/1
  Logical Operator5/1 -> Logical Operator7/2, Switch3/2
  Relational Operator8/1 -> Logical Operator5/1
  Relational Operator9/1 -> Logical Operator5/2
  Constant12/1 -> Relational Operator9/2
  Constant10/1 -> Relational Operator8/2
  Switch1/1 -> signal_debug1/1
  Constant9/1 -> Switch1/1
  Logical Operator4/1 -> Logical Operator7/1, Switch1/2
  Relational Operator6/1 -> Logical Operator4/1
  Relational Operator7/1 -> Logical Operator4/2
  Constant7/1 -> Relational Operator7/2
  Constant6/1 -> Relational Operator6/2
  LPF2/1 -> Relational Operator6/1, Relational Operator10/1, Relational Operator11/1, Relational Operator9/1, Relational Operator8/1, Relational Operator7/1  "IPTd_v_CC"
  ADC to Actual Value/1 -> LPF2/1
  HLd_adc_CC/1 -> ADC to Actual Value/1
  signal_debug/1 -> IPTd_flg_SlowChaCnctSt/1  "IPTd_flg_SlowChaCnctSt"
  Constant2/1 -> IPTd_iflt_CCCnctSt_warn/1  "IPTd_iflt_CCCnctSt_warn"
  Logical Operator7/1 -> Terminator/1
  signal_debug1/1 -> [IPTd_enum_CC], IPTd_enum_CC/1  "IPTd_enum_CC"

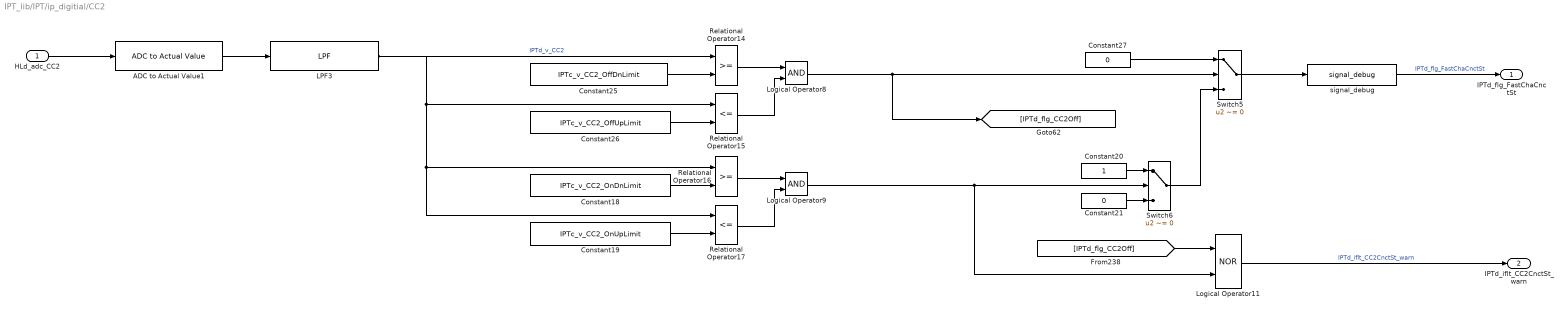
== system IPT_lib/IPT/ip_digitial/CC2 ==
  HLd_adc_CC2 : Inport  OutDataType=fixdt(1, 16)  OutScaling=2^0
  ADC to Actual Value1 : Defined_Functionality/ADC to Actual Value  SystemSampleTime=-1  gain=0.001221  offset=0
      settings: AttributesFormatString=[GAIN=%<gain>]\n[OFFSET=%<offset>]
  Constant18 : Constant  Value=IPTc_v_CC2_OnDnLimit  OutDataType=fixdt(1, 16)  OutScaling=2^0
  Constant19 : Constant  Value=IPTc_v_CC2_OnUpLimit  OutDataType=fixdt(1, 16)  OutScaling=2^0
  Constant20 : Constant  OutDataTypeMode=boolean  OutDataType=fixdt(1, 16)  OutScaling=2^0  OutDataTypeStr=boolean
  Constant21 : Constant  Value=0  OutDataTypeMode=boolean  OutDataType=fixdt(1, 16)  OutScaling=2^0  OutDataTypeStr=boolean
  Constant25 : Constant  Value=IPTc_v_CC2_OffDnLimit  OutDataType=fixdt(1, 16)  OutScaling=2^0
  Constant26 : Constant  Value=IPTc_v_CC2_OffUpLimit  OutDataType=fixdt(1, 16)  OutScaling=2^0
  Constant27 : Constant  Value=0  OutDataTypeMode=boolean  OutDataType=fixdt(1, 16)  OutScaling=2^0  OutDataTypeStr=boolean
  LPF3 : Defined_Functionality/LPF  SystemSampleTime=-1  filter_gain=IPTc_flter_CC2
      settings: AttributesFormatString=[FILTER_GAIN=%<filter_gain>]
  Logical Operator11 : Logic  Operator=NOR  AllPortsSameDT=off  OutDataTypeMode=boolean  LogicDataType=fixdt(0, 8)  OutDataTypeStr=boolean
  Logical Operator8 : Logic  AllPortsSameDT=off  OutDataTypeMode=boolean  LogicDataType=fixdt(0, 8)  OutDataTypeStr=boolean
  Logical Operator9 : Logic  AllPortsSameDT=off  OutDataTypeMode=boolean  LogicDataType=fixdt(0, 8)  OutDataTypeStr=boolean
  Relational Operator14 : RelationalOperator  LogicOutDataTypeMode=boolean  LogicDataType=fixdt(0, 8)  OutDataTypeStr=boolean
  Relational Operator15 : RelationalOperator  Operator=<=  LogicOutDataTypeMode=boolean  LogicDataType=fixdt(0, 8)  OutDataTypeStr=boolean
  Relational Operator16 : RelationalOperator  LogicOutDataTypeMode=boolean  LogicDataType=fixdt(0, 8)  OutDataTypeStr=boolean
  Relational Operator17 : RelationalOperator  Operator=<=  LogicOutDataTypeMode=boolean  LogicDataType=fixdt(0, 8)  OutDataTypeStr=boolean
  Switch5 : Switch  Criteria=u2 ~= 0  OutDataType=fixdt(1, 16)  OutScaling=2^0
  Switch6 : Switch  Criteria=u2 ~= 0  OutDataType=fixdt(1, 16)  OutScaling=2^0
  signal_debug : Defined_Functionality/signal_debug  SystemSampleTime=-1  debug_switch=IPTc_dbgsw_FastChaCnctSt  debug_value=IPTc_dbgval_FastChaCnctSt
      settings: AttributesFormatString=[SWITCH=%<debug_switch>]\n[VALUE=%<debug_value>]
  IPTd_flg_FastChaCnctSt : Outport  OutDataType=fixdt(1, 16)  OutScaling=2^0
  IPTd_iflt_CC2CnctSt_warn : Outport  Port=2  OutDataType=fixdt(1, 16)  OutScaling=2^0
  wires:
  Constant21/1 -> Switch6/3
  Logical Operator11/1 -> IPTd_iflt_CC2CnctSt_warn/1  "IPTd_iflt_CC2CnctSt_warn"
  Switch6/1 -> Switch5/3
  Constant20/1 -> Switch6/1
  Switch5/1 -> signal_debug/1
  Constant27/1 -> Switch5/1
  LPF3/1 -> Relational Operator14/1, Relational Operator15/1, Relational Operator17/1, Relational Operator16/1  "IPTd_v_CC2"
  ADC to Actual Value1/1 -> LPF3/1
  HLd_adc_CC2/1 -> ADC to Actual Value1/1
  signal_debug/1 -> IPTd_flg_FastChaCnctSt/1  "IPTd_flg_FastChaCnctSt"
  [IPTd_flg_CC2Off] -> Logical Operator11/1
  Constant25/1 -> Relational Operator14/2
  Constant26/1 -> Relational Operator15/2
  Relational Operator15/1 -> Logical Operator8/2
  Relational Operator14/1 -> Logical Operator8/1
  Constant18/1 -> Relational Operator16/2
  Constant19/1 -> Relational Operator17/2
  Relational Operator17/1 -> Logical Operator9/2
  Relational Operator16/1 -> Logical Operator9/1
  Logical Operator9/1 -> Switch6/2, Logical Operator11/2
  Logical Operator8/1 -> Switch5/2, [IPTd_flg_CC2Off]
